simulink model "Ejemplo_2"  (R2022a)
settings: Solver=ode4  StartTime=0.0  StopTime=200  FixedStep=0.01  RelTol=1e-3
values from neighbouring files (symbols this model uses):
  b = 1.2    [ParametrosEjemplo2.m]    (also in ParametrosEjemploA_3_2.m = 1000)
  k = 300    [ParametrosEjemplo2.m]    (also in ParametrosEjemploA_3_2.m = [0 0 0 1]*inversa*phiA)
  m = 15    [ParametrosEjemplo2.m]
settings Model: Creator=Anahi Monserrat  LastModifiedBy=Anahi Monserrat

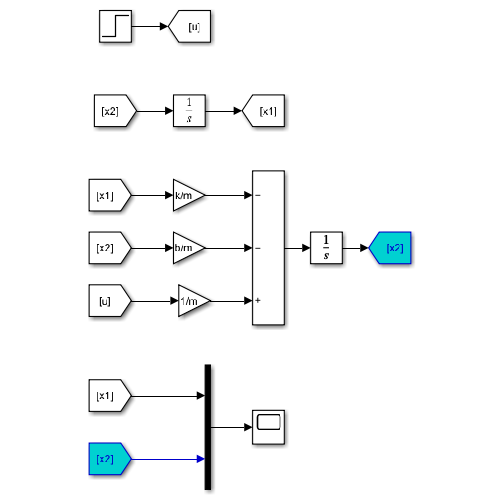
[thumbnail: Simulink's stored preview of the top-level diagram]
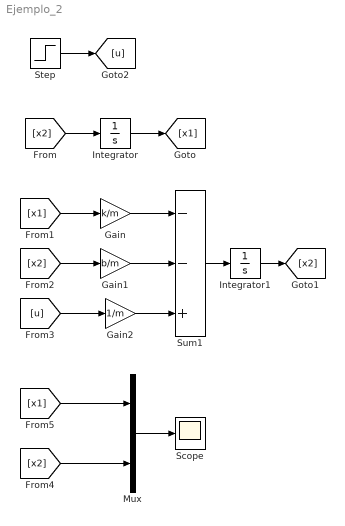
== system Ejemplo_2 ==
  Gain : Gain  Gain=k/m
  Gain1 : Gain  Gain=b/m
  Gain2 : Gain  Gain=1/m
  Integrator : Integrator
  Integrator1 : Integrator
  Mux : Mux  Inputs=2
  Scope : Scope
  Step : Step  SampleTime=0
  Sum1 : Sum  Inputs=--+
  wires:
  [x2] -> Integrator/1
  Integrator/1 -> [x1]
  Integrator1/1 -> [x2]
  Sum1/1 -> Integrator1/1
  [x1] -> Gain/1
  Gain/1 -> Sum1/1
  [x2] -> Gain1/1
  Gain1/1 -> Sum1/2
  Step/1 -> [u]
  [u] -> Gain2/1
  Gain2/1 -> Sum1/3
  Mux/1 -> Scope/1
  [x2] -> Mux/2
  [x1] -> Mux/1
